simulink model "simconsensusbasic"  (Simulink 8.8)
settings: Solver=ode3  StartTime=0.0  StopTime=5  FixedStep=0.001  RelTol=1e-5  EnableMultiTasking=on
values from neighbouring files (symbols this model uses):
  A = [1 0;1 2]    [testparameter.m]
  B = [1;1]    [testparameter.m]
  c = 1    [testparameter.m]
  K = -place(A,B,[-2 -3])    [testparameter.m]
  L = [3 -1 -1 0 -1 ... (first row only)    [testparameter.m]
  N = length(L)    [testparameter.m]
  n = length(A)    [testparameter.m]
  x10 = [0.3 -0.3]    [testparameter.m]
  x20 = [-0.2 0 ]    [testparameter.m]
  x30 = [-0.2 0.2 ]    [testparameter.m]
  x40 = [0 0.1 ]    [testparameter.m]
  x50 = [0.2 0]    [testparameter.m]
settings Model: Creator=Moh3n  LastModifiedBy=The HopePower
settings SolverCC: ShapePreserveControl=EnableAll  ZeroCrossAlgorithm=Adaptive
settings OptimizationCC: ExpressionDepthLimit=2147483647
settings DebuggingCC: SolverPrmCheckMsg=warning
settings ConfigComp: CovSFcnEnable=off

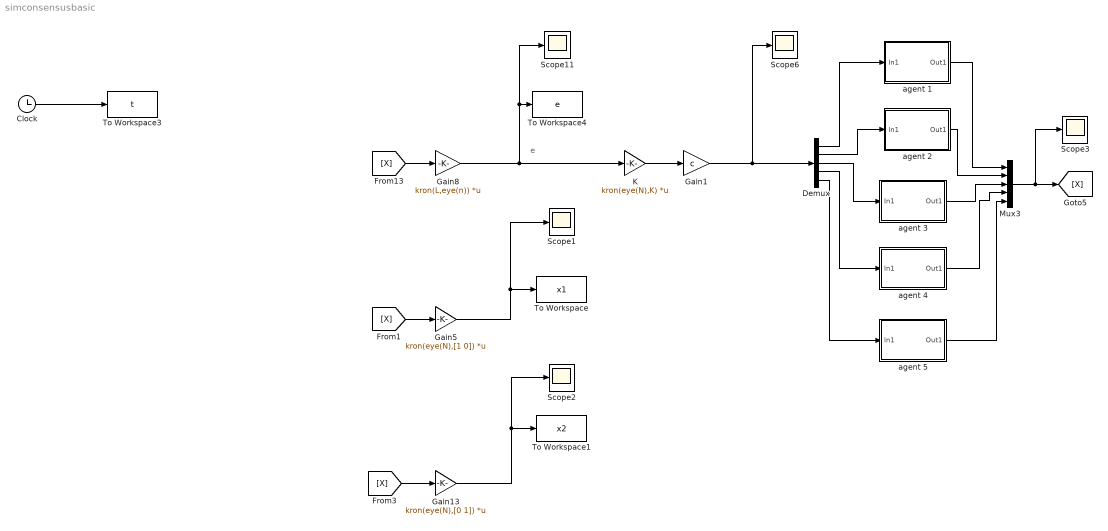
== system simconsensusbasic ==
  note: e
  Clock : Clock
  Demux : Demux  Outputs=5
  Gain1 : Gain  Gain=c
  Gain13 : Gain  Gain=kron(eye(N),[0 1])  Multiplication=Matrix(K*u)
  Gain5 : Gain  Gain=kron(eye(N),[1 0])  Multiplication=Matrix(K*u)
  Gain8 : Gain  Gain=kron(L,eye(n))  Multiplication=Matrix(K*u)
  K : Gain  Gain=kron(eye(N),K)  Multiplication=Matrix(K*u)
  Mux3 : Mux  Inputs=5
  Scope{1..3,6,11} (5 alike) : Scope
  To Workspace : ToWorkspace  VariableName=x1  SampleTime=-1
  To Workspace1 : ToWorkspace  VariableName=x2  SampleTime=-1
  To Workspace3 : ToWorkspace  VariableName=t  SampleTime=-1
  To Workspace4 : ToWorkspace  VariableName=e  SampleTime=-1
  agent 1 : Subsystem
  agent 2 : Subsystem
  agent 3 : Subsystem
  agent 4 : Subsystem
  agent 5 : Subsystem
  wires:
  [X] -> Gain8/1
  Mux3/1 -> [X], Scope3/1
  Demux/2 -> agent 2/1(In1)
  Demux/3 -> agent 3/1(In1)
  agent 1/1(Out1) -> Mux3/1
  agent 2/1(Out1) -> Mux3/2
  agent 3/1(Out1) -> Mux3/3
  agent 4/1(Out1) -> Mux3/4
  Demux/1 -> agent 1/1(In1)
  Demux/4 -> agent 4/1(In1)
  [X] -> Gain5/1
  Gain5/1 -> Scope1/1, To Workspace/1
  [X] -> Gain13/1
  Gain13/1 -> Scope2/1, To Workspace1/1
  Gain8/1 -> Scope11/1, To Workspace4/1, K/1
  agent 5/1(Out1) -> Mux3/5
  Demux/5 -> agent 5/1(In1)
  Gain1/1 -> Demux/1, Scope6/1
  Clock/1 -> To Workspace3/1
  K/1 -> Gain1/1

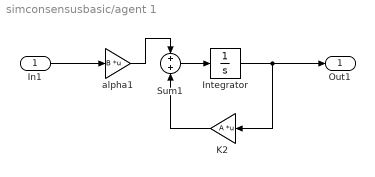
== system simconsensusbasic/agent 1 ==
  In1 : Inport
  Integrator : Integrator  InitialCondition=x10
  K2 : Gain  Gain=A  Multiplication=Matrix(K*u)
  Sum1 : Sum
  alpha1 : Gain  Gain=B  Multiplication=Matrix(K*u)
  Out1 : Outport
  wires:
  In1/1 -> alpha1/1
  alpha1/1 -> Sum1/1
  Sum1/1 -> Integrator/1
  Integrator/1 -> K2/1, Out1/1
  K2/1 -> Sum1/2

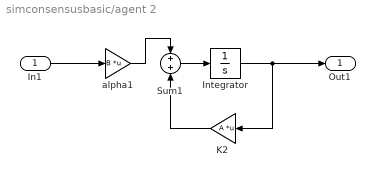
== system simconsensusbasic/agent 2 ==
  In1 : Inport
  Integrator : Integrator  InitialCondition=x20
  K2 : Gain  Gain=A  Multiplication=Matrix(K*u)
  Sum1 : Sum
  alpha1 : Gain  Gain=B  Multiplication=Matrix(K*u)
  Out1 : Outport
  wires:
  In1/1 -> alpha1/1
  Sum1/1 -> Integrator/1
  Integrator/1 -> K2/1, Out1/1
  alpha1/1 -> Sum1/1
  K2/1 -> Sum1/2

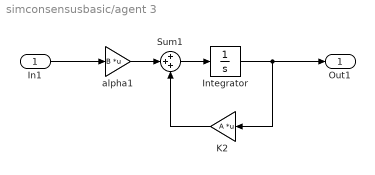
== system simconsensusbasic/agent 3 ==
  In1 : Inport
  Integrator : Integrator  InitialCondition=x30
  K2 : Gain  Gain=A  Multiplication=Matrix(K*u)
  Sum1 : Sum  Inputs=+++
  alpha1 : Gain  Gain=B  Multiplication=Matrix(K*u)
  Out1 : Outport
  wires:
  In1/1 -> alpha1/1
  alpha1/1 -> Sum1/2
  K2/1 -> Sum1/3
  Sum1/1 -> Integrator/1
  Integrator/1 -> K2/1, Out1/1

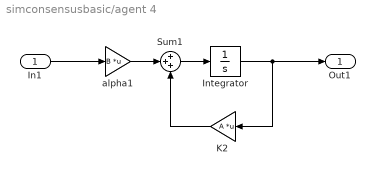
== system simconsensusbasic/agent 4 ==
  In1 : Inport
  Integrator : Integrator  InitialCondition=x40
  K2 : Gain  Gain=A  Multiplication=Matrix(K*u)
  Sum1 : Sum  Inputs=+++
  alpha1 : Gain  Gain=B  Multiplication=Matrix(K*u)
  Out1 : Outport
  wires:
  In1/1 -> alpha1/1
  alpha1/1 -> Sum1/2
  K2/1 -> Sum1/3
  Sum1/1 -> Integrator/1
  Integrator/1 -> K2/1, Out1/1

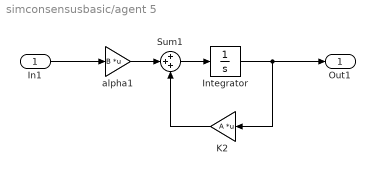
== system simconsensusbasic/agent 5 ==
  In1 : Inport
  Integrator : Integrator  InitialCondition=x50
  K2 : Gain  Gain=A  Multiplication=Matrix(K*u)
  Sum1 : Sum  Inputs=+++
  alpha1 : Gain  Gain=B  Multiplication=Matrix(K*u)
  Out1 : Outport
  wires:
  In1/1 -> alpha1/1
  alpha1/1 -> Sum1/2
  K2/1 -> Sum1/3
  Sum1/1 -> Integrator/1
  Integrator/1 -> K2/1, Out1/1
